simulink model "fluidMechanicsSim"  (R2025b)
settings: Solver=VariableStepAuto  StartTime=0.0  StopTime=10  RelTol=1e-3
undefined symbols (not defined in the file or in its folder): constantsSTADPOLE
settings Model: Creator=Eric  LastModifiedBy=Eric

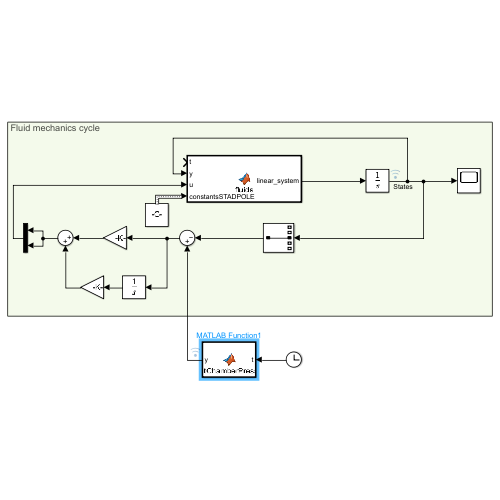
[thumbnail: Simulink's stored preview of the top-level diagram]
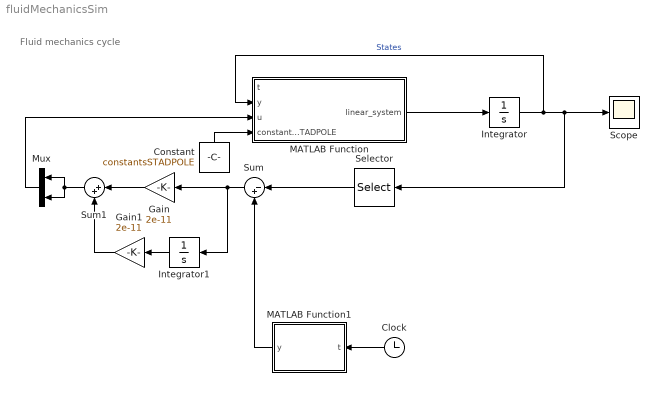
== system fluidMechanicsSim ==
  note: Fluid mechanics cycle
  Clock : Clock
  Constant : Constant  Value=constantsSTADPOLE  OutDataTypeStr=Bus: slBus1
  Gain : Gain  Gain=2e-11
  Gain1 : Gain  Gain=2e-11
  Integrator : Integrator  InitialCondition=[1e-6; 1e-6; 1e5; 1e5; 1e5]
  Integrator1 : Integrator
  MATLAB Function : MATLAB Function  TreatAsAtomicUnit=on
  MATLAB Function1 : MATLAB Function  TreatAsAtomicUnit=on
  Mux : Mux  Inputs=2
  Scope : Scope
      settings: ActiveDisplayYMinimum=-508618.55034345371  ActiveDisplayYMaximum=4.577570953091085E+6
  Selector : Selector  InputPortWidth=5  IndexOptions=Index vector (dialog)  Indices=3  OutputSizes=1
  Sum : Sum  Inputs=|-+
  Sum1 : Sum  Inputs=|++
  wires:
  Integrator/1 -> MATLAB Function/2(y), Selector/1, Scope/1  "States"
  MATLAB Function/1(linear_system) -> Integrator/1
  Selector/1 -> Sum/1
  MATLAB Function1/1(y) -> Sum/2
  Sum/1 -> Integrator1/1, Gain/1
  Mux/1 -> MATLAB Function/3(u)
  Integrator1/1 -> Gain1/1
  Gain1/1 -> Sum1/2
  Gain/1 -> Sum1/1
  Sum1/1 -> Mux/1, Mux/2
  Clock/1 -> MATLAB Function1/1(t)
  Constant/1 -> MATLAB Function/4(constantsSTADPOLE)

== matlab function fluidMechanicsSim/MATLAB Function1 ==
  data: t input; y output
function y = inputChamberPressure(t)

% y = 300000*tanh(t) + 2E06;
y = 2E06;

== matlab function fluidMechanicsSim/MATLAB Function ==
  data: t input; linear_system output; y input; u input; constantsSTADPOLE input
function linear_system = fluids(t,y,u, constantsSTADPOLE)
   
    linear_system = fluidMechanics(t,y,u, constantsSTADPOLE);
end
